simulink model "Set_Spd_Fdfwd_Deccel"  (R2024a)
settings: Solver=FixedStepDiscrete  StartTime=0.0  StopTime=10.0  RelTol=1e-3
settings Model: Creator=darkh  LastModifiedBy=darkh
settings OptimizationCC: ZeroExternalMemoryAtStartup=off  ZeroInternalMemoryAtStartup=off
settings RTWCC: Description=Generate an RTMaps component embedding the model  SystemTargetFile=rtmaps.tlc  TemplateMakefile=rtmaps_default_tmf  PostCodeGenCommand=rtmaps_post_code_generation(buildInfo)  RetainRTWFile=on  TargetLang=C++
settings STFCustomTargetCC: TargetLangStandard=C++11 (ISO)  ModelReferenceCompliant=off  ConcurrentExecutionCompliant=on  CombineOutputUpdateFcns=on  CodeInterfacePackaging=C++ class  CPPClassGenCompliant=on  GRTInterface=off  UseToolchainInfoCompliant=off  SystemTargetFile=rtmaps.tlc
settings GRTTargetCC: TargetLangStandard=C++11 (ISO)  ModelReferenceCompliant=off  ParMdlRefBuildCompliant=off  CompOptLevelCompliant=off  MatFileLogging=off  CodeInterfacePackaging=C++ class  UseToolchainInfoCompliant=off

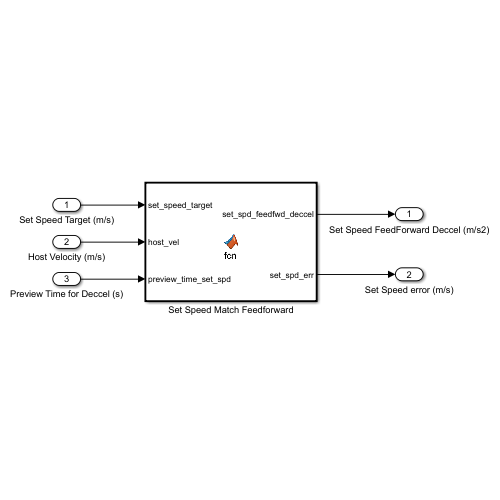
[thumbnail: Simulink's stored preview of the top-level diagram]
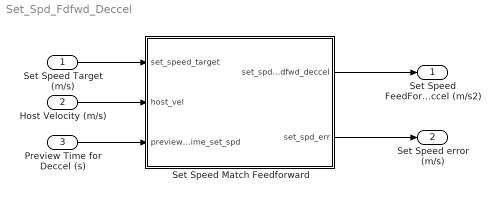
== system Set_Spd_Fdfwd_Deccel ==
  Set Speed Target (m/s) : Inport
  Host Velocity (m/s) : Inport  Port=2
  Preview Time for Deccel (s) : Inport  Port=3
  Set Speed Match Feedforward : MATLAB Function  TreatAsAtomicUnit=on
  Set Speed FeedForward Deccel (m/s2) : Outport
  Set Speed error (m/s) : Outport  Port=2
  wires:
  Set Speed Target (m/s)/1 -> Set Speed Match Feedforward/1(set_speed_target)
  Host Velocity (m/s)/1 -> Set Speed Match Feedforward/2(host_vel)
  Preview Time for Deccel (s)/1 -> Set Speed Match Feedforward/3(preview_time_set_spd)
  Set Speed Match Feedforward/1(set_spd_feedfwd_deccel) -> Set Speed FeedForward Deccel (m/s2)/1
  Set Speed Match Feedforward/2(set_spd_err) -> Set Speed error (m/s)/1

== matlab function Set_Spd_Fdfwd_Deccel/Set Speed Match Feedforward ==
  data: set_speed_target input; set_spd_feedfwd_deccel output; host_vel input; preview_time_set_spd input; set_spd_err output
function [set_spd_feedfwd_deccel, set_spd_err] = fcn(set_speed_target, host_vel, preview_time_set_spd)
% This function determines the feedforward slowing down effect for host if
% the vehicle ever exceeds the set speed maximum/driver set speed/speed target set by AIN feature
% inputs are set_speed_target [m/s] which is speed maximum value; host_vel which is host velocity feedback [m/s]; 
% preview_time [secs] is how quickly want vehicle to slow down to bring below/at set speed maximum

set_spd_err = set_speed_target - host_vel; % if over set speed limit this value will be negative
if set_spd_err < 0.0
    set_spd_feedfwd_deccel = set_spd_err/preview_time_set_spd;
    return;
end

set_spd_feedfwd_deccel = 0.0;
